simulink model "Kundur_BESS_STA_Nov14_2021a_v2_2021a"  (R2023a)
settings: Solver=VariableStepAuto  StartTime=0.0  StopTime=3  FixedStep=Ts  MaxStep=1e-5  MinStep=1e-20  RelTol=1e-3  EnableMultiTasking=on
PreLoadFcn:
  | Ts=50e-6;
PostLoadFcn:
  | Ts=50e-6;
InitFcn:
  | Ts=50e-6;
values from neighbouring files (symbols this model uses):
  current_K_den = [1 -1.95396088137 0.953960881373]    [param_cntrl_v2.mat]
  current_K_num = [292.549944556 -582.765243791 290.215658722]    [param_cntrl_v2.mat]
  flt_den = [1 -1.99914493247 0.999500180349]    [param_cntrl_v2.mat]
  flt_num = [0.000249925443627 3.12366678454e-08 -0.000249894206959]    [param_cntrl_v2.mat]
  flt_rocof_den = [1 -3.94812243331 5.84544117496 -3.84650440967 0.949185710471]    [param_cntrl_v2.mat]
  flt_rocof_num = [2.65341753303e-09 1.06136701321e-08 1.59205051982e-08 1.06136701321e-08 2.65341753303e-09]    [param_cntrl_v2.mat]
  pll_K_den = [1 -1.95396088137 0.953960881373]    [param_cntrl_v2.mat]
  pll_K_num = [1047.77474974 -2078.89023245 1031.12061217]    [param_cntrl_v2.mat]
  sampling_k = 5e-05    [param_cntrl_v2.mat]
undefined symbols (not defined in the file or in its folder): Ad2, Ad4, Bd2, Bd4, Cd2, Cd4, D1, Delta, flt_rocof_a_den, flt_rocof_a_num, flt_rocof_b_den, flt_rocof_b_num, Gd2, Gd4, Kd2, Kd4, L, R
libraries: spsThreePhaseVIMeasurementLib x15, spsLoadFlowBusLib x12, spsSeriesRLCBranchLib x11, spsThreePhaseSeriesRLCLoadLib x11, spsThreePhaseTransformerTwoWindingsLib x8, spsThreePhaseSeriesRLCBranchLib x8, spsabctoAlphaBetaZeroLib x8, spsGenericPowerSystemStabilizerLib x8, spsPowerPositiveSequenceLib x7, spsThreePhaseParallelRLCLoadLib x6, spsPLL3phLib x6, spsGroundLib x6
(part 1 of 4)
Description:
  | Model of a simple control system for use iin training.
settings Model: Creator=Paul Baracos  LastModifiedBy=juang
settings SolverCC: MaxConsecutiveZCs=10000  MaxConsecutiveMinStep=10  SolverJacobianMethodControl=FullAnalytical
settings DataIOCC: LimitDataPoints=on  SaveFormat=Array  SignalLoggingSaveFormat=ModelDataLogs  SaveOutput=off  SaveTime=off  ReturnWorkspaceOutputs=off  SignalLoggingName=sigsOut
settings OptimizationCC: BlockReduction=off  BooleanDataType=off  OptimizeBlockIOStorage=off  BufferReuse=off  GlobalBufferReuse=off  ExpressionFolding=off  LocalBlockOutputs=off  InitFltsAndDblsToZero=on  LifeSpan=inf  OptimizeDataStoreBuffers=off  BusAssignmentInplaceUpdate=off
settings DebuggingCC: SaveWithParameterizedLinksMsg=none  UnderspecifiedInitializationDetection=Classic  MergeDetectMultiDrivingBlocksExec=none  SignalResolutionControl=TryResolveAllWithWarning  MultiTaskDSMMsg=warning  MultiTaskCondExecSysMsg=none  FcnCallInpInsideContextMsg=warning  UnconnectedInputMsg=warning  UnconnectedOutputMsg=warning  UnconnectedLineMsg=warning  SFUnexpectedBacktrackingDiag=warning  SFNoUnconditionalDefaultTransitionDiag=warning  ArithmeticOperatorsInVariantConditions=warning
settings HardwareCC: ProdBitPerPointer=32  ProdBitPerSizeT=32  ProdBitPerPtrDiffT=32  ProdLargestAtomicFloat=None  ProdIntDivRoundTo=Undefined  ProdEndianess=Unspecified  ProdWordSize=32  ProdHWDeviceType=32-bit Generic  TargetBitPerPointer=64  TargetBitPerSizeT=64  TargetBitPerPtrDiffT=64  TargetLongLongMode=on  TargetIntDivRoundTo=Zero  TargetEndianess=LittleEndian  TargetWordSize=64  TargetHWDeviceType=MATLAB Host  ProdEqTarget=off
settings ModelReferenceCC: EnableRefExpFcnMdlSchedulingChecks=on  PropagateSignalLabelsOutOfModel=off
settings SFSimCC: SimUseLocalCustomCode=off  CustomCodeUndefinedFunction=UseInterfaceOnly
settings RTWCC: RTWUseLocalCustomCode=off
settings CodeAppCC: StateflowObjectComments=on
settings GRTTargetCC: TargetFcnLib=ansi_tfl_tmw.mat  TargetLangStandard=C89/C90 (ANSI)  CombineOutputUpdateFcns=off  GRTInterface=on
settings ConfigComp: CovMetricSettings=dw  CovSaveCumulativeToWorkspaceVar=on  CovSaveSingleToWorkspaceVar=on  CovExternalEMLEnable=off
settings SimscapeCC: SimscapeNormalizeSystem=off

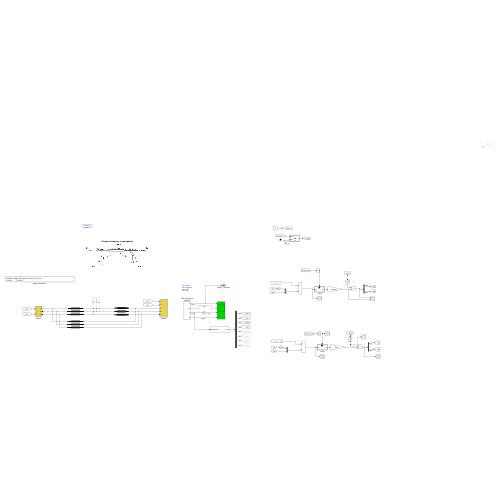
[thumbnail: Simulink's stored preview of the top-level diagram]
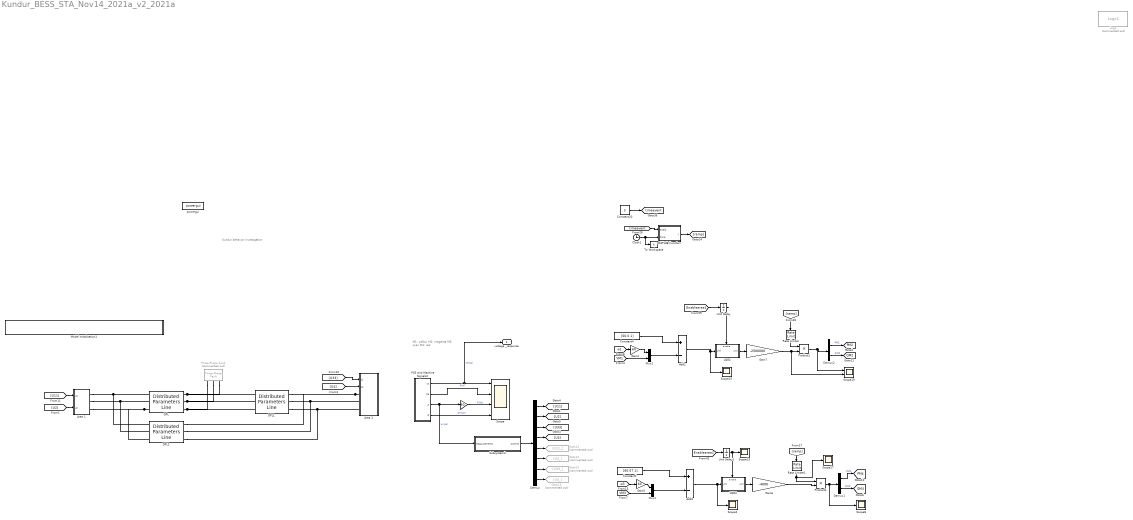
== system Kundur_BESS_STA_Nov14_2021a_v2_2021a ==
  note: Kundur behavior investigation
  note: M1: yellow
      | M2: magenta
      | M3: cyan
      | M4: red
  " " : Gain  Gain=60  SaturateOnIntegerOverflow=on  OutDataTypeStr=Inherit: Same as input  ParamDataTypeStr=Inherit: Same as input
  Add2 : Sum  Inputs=+-
  Add3 : Sum  Inputs=+-
  Area 1 : Subsystem
  Area 2 : Subsystem
  Clock1 : Clock
  Constant1 : Constant  Value=[60.07 1]
  Constant20 : Constant  Value=3
  Constant4 : Constant  Value=[60.0 1]
  DPL : spsDistributedParametersLineLib/Distributed Parameters Line  Phases=3  Length=110  Frequency=60  Resistance=[0.0001*529 1.61]  Inductance=[0.001*529/(377) 0.0061]  Capacitance=[0.00175/529/(377) 5.2489e-9]  x1=[-0.00065 2.34503898169386e-05 162037.072789035 -201564.621940964;-0.0006 2.16068678041118e-05 165807.483999355 -198474.662134838;-0.00055 1.97556689740379e-05 169518.984600121 -195314.185226316;-0.0005 1.78974510488464e-05 173170.255912845 -192084.314117795;-0.00045 1.60328742445181e-05 176760.000658212 -188786.1963671;-0.0004 1.41626010363132e-05 180286.94341701 -185421.003779764;-0.00035 1.22872959233969e-05 183749.831083269 -181989.931992688;-0.0003 1.04076251927465e-05 187147.433309491 -178494.200049342;-0.00025 8.52425668242225e-06 190478.542943782 -174935.04996664;-0.0002 6.63785954428797e-06 193741.976458752 -171313.746293659;-0.00015 4.74910400626456e-06 196936.574372011 -167631.57566235;-0.0001 2.85866113420113e-06 200061.201658132 -163889.846330406;-5e-05 9.67202593448582e-07 203114.74815192 -160089.887716441]  x2=[-0.00065 3.04897605546982e-05 118816.066831868 -195960.878256138;-0.0006 2.90157468011296e-05 122488.530340616 -193686.56156247;-0.00055 2.75314238908845e-05 126117.474257778 -191343.428955741;-0.0005 2.60373191968251e-05 129701.60923686 -188932.312939808;-0.00045 2.45339635672348e-05 133239.661851769 -186454.070172711;-0.0004 2.30218911372104e-05 136730.375049258 -183909.581162304;-0.00035 2.15016391388865e-05 140172.50859555 -181299.749953418;-0.0003 1.99737477105591e-05 143564.839516987 -178625.503806653;-0.00025 1.84387597047774e-05 146906.162534544 -175887.792868933;-0.0002 1.6897220495471e-05 150195.290492063 -173087.589835917;-0.00015 1.53496777841807e-05 153431.054778043 -170225.889606408;-0.0001 1.3796681405463e-05 156612.30574084 -167303.708928874;-5e-05 1.22387831315364e-05 159737.913097136 -164322.086040193]  x3=[-0.00065 -7.70603438254632e-09 386.387902520665 214.266648693801;-0.0006 -8.20654088038672e-09 382.28069114739 221.511346722587;-0.00055 -8.70413163332872e-09 378.037657264824 228.677342824636;-0.0005 -9.19862984974715e-09 373.660308402703 235.762090955653;-0.00045 -9.68985983678033e-09 369.150199812235 242.763073938362;-0.0004 -1.01776470627529e-08 364.508933913525 249.677804356846;-0.00035 -1.06618182191862e-08 359.738159726248 256.503825440312;-0.0003 -1.11422012823736e-08 354.839572283756 263.238711935973;-0.00025 -1.16186255745004e-08 349.814912030842 269.880070970725;-0.0002 -1.2090921824284e-08 344.665964205369 276.425542901327;-0.00015 -1.25589222271158e-08 339.394558203981 282.872802152769;-0.0001 -1.30224605046811e-08 334.00256693213 289.219558044538;-5e-05 -1.3481371964037e-08 328.491906138641 295.463555604487]  x4=[-0.00065 6.9623199876992e-08 236.382256048156 -1248.37836597241;-0.0006 6.7501778785042e-08 259.870303302539 -1243.70107133658;-0.00055 6.53563746325074e-08 283.266019875563 -1238.58189563215;-0.0005 6.3187749671268e-08 306.561093380529 -1233.02265767785;-0.00045 6.09966744034463e-08 329.747247188744 -1227.02533264446;-0.0004 5.87839273076519e-08 352.816243370164 -1220.592051353;-0.00035 5.65502945623917e-08 375.75988562029 -1213.7250995177;-0.0003 5.42965697667444e-08 398.57002217228 -1206.42691693383;-0.00025 5.20235536583985e-08 421.238548693231 -1198.70009661092;-0.0002 4.97320538291541e-08 443.757411163608 -1190.54738385143;-0.00015 4.74228844379892e-08 466.118608738802 -1181.97167527539;-0.0001 4.50968659217932e-08 488.314196591789 -1172.97601779123;-5e-05 4.27548247038692e-08 510.336288735894 -1163.56360751321]  x5=0.000622431770558027  V1=[0 0 0 8.852e-11 2.458e+05 2.458e+05;0 0 0 377 377 377;1.571 1.571 1.571 -1.64 0.7159 -0.8549]  V2=[0 0 0 1.627e-10 2.245e+05 2.245e+05;0 0 0 377 377 377;1.571 1.571 1.571 -1.342 0.5232 -1.048]  I1=[0 0 0 6.584e-13 354.7 354.2;0 0 0 377 377 377;1.571 1.571 1.571 -2.457 2.767 1.197]  I2=[0 0 0 4.221e-13 1404 1403;0 0 0 377 377 377;1.571 1.571 1.571 -0.7538 0.3476 -1.223]  nHarmo=2  Measurements=None  Decoupling=off  VsMag0=0  VrMag0=0  VsAngle0=0  VrAngle0=0  IsMag0=0  IrMag0=0  IsAngle0=0  IrAngle0=0
  DPL1 : spsDistributedParametersLineLib/Distributed Parameters Line  Phases=3  Length=110  Frequency=60  Resistance=[0.0001*529 1.61]  Inductance=[0.001*529/(377) 0.0061]  Capacitance=[0.00175/529/(377) 5.2489e-9]  x1=[-0.00065 3.04897737893273e-05 118816.066831868 -195960.878256138;-0.0006 2.90157601664698e-05 122488.530340616 -193686.56156247;-0.00055 2.75314373821871e-05 126117.474257778 -191343.428955741;-0.0005 2.60373328092966e-05 129701.60923686 -188932.312939808;-0.00045 2.45339772960389e-05 133239.661851769 -186454.070172711;-0.0004 2.30219049774693e-05 136730.375049258 -183909.581162304;-0.00035 2.15016530856827e-05 140172.50859555 -181299.749953418;-0.0003 1.99737617589375e-05 143564.839516987 -178625.503806653;-0.00025 1.84387738497467e-05 146906.162534544 -175887.792868933;-0.0002 1.68972347320055e-05 150195.290492063 -173087.589835917;-0.00015 1.53496921072222e-05 153431.054778043 -170225.889606408;-0.0001 1.37966958099226e-05 156612.30574084 -167303.708928874;-5e-05 1.22387976122963e-05 159737.913097136 -164322.086040193]  x2=[-0.00065 3.28792055379406e-05 73497.1281809996 -185964.418906558;-0.0006 3.18342069047249e-05 76989.2205617754 -184546.068621456;-0.00055 3.07778977293782e-05 80453.9590390789 -183062.149996912;-0.0005 2.97106533135209e-05 83890.1126078269 -181513.190262145;-0.00045 2.86328528440121e-05 87296.4604190179 -179899.739755175;-0.0004 2.75448792582265e-05 90671.7922134945 -178222.371727283;-0.00035 2.64471191079986e-05 94014.908751942 -176481.682139344;-0.0003 2.53399624222828e-05 97324.6222409731 -174678.289450079;-0.00025 2.42238025685775e-05 100599.756755145 -172812.834396324;-0.0002 2.30990361131641e-05 103839.148654759 -170885.979765376;-0.00015 2.19660626802085e-05 107041.646999298 -168898.410159511;-0.0001 2.08252848097767e-05 110206.11395635 -166850.831752747;-5e-05 1.96771078148139e-05 113331.425205873 -164743.972039941]  x3=[-0.00065 -1.95769407602966e-08 351.42047903309 278.927488837443;-0.0006 -1.98750329311255e-08 346.100716190805 285.501615062663;-0.00055 -2.01660635973912e-08 340.657985412057 291.974303923501;-0.0005 -2.04499293572839e-08 335.094220473176 298.343255704425;-0.00045 -2.07265293546507e-08 329.41139815335 304.606207547194;-0.0004 -2.09957653148295e-08 323.611537532293 310.760934254839;-0.00035 -2.12575415795659e-08 317.696699272864 316.805249082269;-0.0003 -2.15117651409993e-08 311.668984888935 322.737004513205;-0.00025 -2.17583456747089e-08 305.530535998722 328.554093023188;-0.0002 -2.19971955718053e-08 299.28353356389 334.254447828369;-0.00015 -2.22282299700572e-08 292.930197114655 339.836043619829;-0.0001 -2.24513667840431e-08 286.472783961208 345.29689728316;-5e-05 -2.26665267343154e-08 279.913588391693 350.635068603058]  x4=[-0.00065 8.49527153453681e-08 55.1658815479513 -1258.43087921918;-0.0006 8.33025259626403e-08 78.8755823413983 -1257.16743857369;-0.00055 8.16227395890926e-08 102.557259016015 -1255.45733232342;-0.0005 7.99139530448253e-08 126.202497584841 -1253.30116806099;-0.00045 7.81767734535609e-08 149.802897007204 -1250.69971186129;-0.0004 7.64118180269363e-08 173.350072173564 -1247.65388800932;-0.00035 7.46197138452107e-08 196.835656884708 -1244.16477867178;-0.0003 7.28010976344665e-08 220.251306824217 -1240.23362351263;-0.00025 7.09566155403837e-08 243.588702523164 -1235.86181925256;-0.0002 6.90869228986678e-08 266.83955231598 -1231.05091917281;-0.00015 6.71926840022114e-08 289.995595286447 -1225.80263256327;-0.0001 6.5274571865075e-08 313.048604202757 -1220.11882411519;-5e-05 6.33332679833675e-08 335.990388440611 -1214.00151325863]  x5=0.000622431770558027  V1=[0 0 0 1.627e-10 2.245e+05 2.245e+05;0 0 0 377 377 377;1.571 1.571 1.571 -1.342 0.5232 -1.048]  V2=[0 0 0 2.11e-10 2.083e+05 2.083e+05;0 0 0 377 377 377;1.571 1.571 1.571 -0.9957 0.2975 -1.273]  I1=[0 0 0 5.999e-13 365.5 365;0 0 0 377 377 377;1.571 1.571 1.571 -1.212 2.93 1.359]  I2=[0 0 0 3.403e-13 1391 1390;0 0 0 377 377 377;1.571 1.571 1.571 2.907 0.203 -1.368]  nHarmo=2  Measurements=None  Decoupling=off  VsMag0=0  VrMag0=0  VsAngle0=0  VrAngle0=0  IsMag0=0  IrMag0=0  IsAngle0=0  IrAngle0=0
  DPL2 : spsDistributedParametersLineLib/Distributed Parameters Line  Phases=3  Length=220  Frequency=60  Resistance=[0.0001*529 1.61]  Inductance=[0.001*529/(377) 0.0061]  Capacitance=[0.00175/529/(377) 5.2489e-9]  x1=[-0.00125 4.47388675144062e-05 112704.215489258 -232770.393652631;-0.0012 4.30375462134881e-05 117071.56879016 -230604.733707614;-0.00115 4.13209338773288e-05 121397.32712012 -228357.140998763;-0.0011 3.95896404101173e-05 125679.953557802 -226028.414085065;-0.00105 3.78442809321789e-05 129917.926506425 -223619.380352103;-0.001 3.60854755614253e-05 134109.74023438 -221130.895718092;-0.00095 3.43138491930299e-05 138253.905410208 -218563.844329773;-0.0009 3.25300312774057e-05 142348.949631757 -215919.138248282;-0.00085 3.07346555965643e-05 146393.417949313 -213197.717125095;-0.0008 2.8928360038936e-05 150385.873382542 -210400.54786818;-0.00075 2.71117863727318e-05 154324.897431037 -207528.624298454;-0.0007 2.52855800179252e-05 158209.090578311 -204582.966796687;-0.00065 2.34503898169386e-05 162037.072789035 -201564.621940964;-0.0006 2.16068678041118e-05 165807.483999355 -198474.662134838;-0.00055 1.97556689740379e-05 169518.984600121 -195314.185226316;-0.0005 1.78974510488464e-05 173170.255912845 -192084.314117795;-0.00045 1.60328742445181e-05 176760.000658212 -188786.1963671;-0.0004 1.41626010363132e-05 180286.94341701 -185421.003779764;-0.00035 1.22872959233969e-05 183749.831083269 -181989.931992688;-0.0003 1.04076251927465e-05 187147.433309491 -178494.200049342;-0.00025 8.52425668242225e-06 190478.542943782 -174935.04996664;-0.0002 6.63785954428797e-06 193741.976458752 -171313.746293659;-0.00015 4.74910400626456e-06 196936.574372011 -167631.57566235;-0.0001 2.85866113420113e-06 200061.201658132 -163889.846330406;-5e-05 9.67202593448582e-07 203114.74815192 -160089.887716441]  x2=[-0.00125 4.44062308903789e-05 29918.4277641747 -197710.675173221;-0.0012 4.35246405678654e-05 33639.6583650254 -197111.626699133;-0.00115 4.26275861478058e-05 37348.9369554381 -196442.54540265;-0.0011 4.17153863493642e-05 41044.945646392 -195703.669005169;-0.00105 4.07883652727854e-05 44726.371263598 -194895.260025957;-0.001 3.98468522842439e-05 48391.905814064 -194017.605688875;-0.00095 3.88911818988212e-05 52040.246950818 -193071.017820329;-0.0009 3.79216936616548e-05 55670.0984356262 -192055.832738482;-0.00085 3.6938732027299e-05 59280.1705995399 -190972.41113376;-0.0008 3.59426462373421e-05 62869.1808011092 -189821.137940699;-0.00075 3.49337901963222e-05 66435.8538820988 -188602.422201184;-0.0007 3.39125223459869e-05 69978.9226205463 -187316.696919113;-0.00065 3.28792055379406e-05 73497.1281809996 -185964.418906558;-0.0006 3.18342069047249e-05 76989.2205617754 -184546.068621456;-0.00055 3.07778977293782e-05 80453.9590390789 -183062.149996912;-0.0005 2.97106533135209e-05 83890.1126078269 -181513.190262145;-0.00045 2.86328528440121e-05 87296.4604190179 -179899.739755175;-0.0004 2.75448792582265e-05 90671.7922134945 -178222.371727283;-0.00035 2.64471191079986e-05 94014.908751942 -176481.682139344;-0.0003 2.53399624222828e-05 97324.6222409731 -174678.289450079;-0.00025 2.42238025685775e-05 100599.756755145 -172812.834396324;-0.0002 2.30990361131641e-05 103839.148654759 -170885.979765376;-0.00015 2.19660626802085e-05 107041.646999298 -168898.410159511;-0.0001 2.08252848097767e-05 110206.11395635 -166850.831752747;-5e-05 1.96771078148139e-05 113331.425205873 -164743.972039941]  x3=[-0.00125 -2.93418450150669e-09 420.706842786539 123.303837466321;-0.0012 -3.36724177725915e-09 418.308051458368 131.211559530522;-0.00115 -3.79910268804167e-09 415.760637271337 139.072662752401;-0.0011 -4.229613795729e-09 413.065505309576 146.884354119415;-0.00105 -4.65862214177452e-09 410.22361314064 154.643858174818;-0.001 -5.08597530155564e-09 407.235970475282 162.348418003767;-0.00095 -5.51152143852959e-09 404.103638808717 169.995296212839;-0.0009 -5.93510935818019e-09 400.82773104347 177.58177590262;-0.00085 -6.35658856173656e-09 397.409411093972 185.105161633;-0.0008 -6.77580929964459e-09 393.849893473024 192.562780380851;-0.00075 -7.19262262477226e-09 390.150442860288 199.951982489743;-0.0007 -7.60688044532988e-09 386.312373652951 207.270142611352;-0.00065 -8.01843557748633e-09 382.337049498727 214.514660638232;-0.0006 -8.42714179766283e-09 378.225882811359 221.682962627624;-0.00055 -8.83285389448545e-09 373.980334268796 228.772501715965;-0.0005 -9.23542772037803e-09 369.601912294218 235.780759023772;-0.00045 -9.63472024277714e-09 365.092172520105 242.705244550597;-0.0004 -1.00305895949509e-08 360.452717235525 249.543498059702;-0.00035 -1.04228951264033e-08 355.68519481685 256.293089952178;-0.0003 -1.08114974528472e-08 350.791299142093 262.951622130164;-0.00025 -1.11962585057263e-08 345.772768989086 269.516728848881;-0.0002 -1.15770415812707e-08 340.631387417694 275.986077557175;-0.00015 -1.19537113890666e-08 335.368981136309 282.357369726252;-0.0001 -1.23261341001251e-08 329.987419852826 288.628341666344;-5e-05 -1.26941773944301e-08 324.488615610343 294.79676533098]  x4=[-0.00125 9.3026611658606e-08 -227.277448411085 -1227.94404256492;-0.0012 9.1902598207341e-08 -204.092223618631 -1232.0096275895;-0.00115 9.0745932200538e-08 -180.834485830935 -1235.63748545975;-0.0011 8.95570245961215e-08 -157.512498411488 -1238.82632721505;-0.00105 8.83362978073024e-08 -134.134547551369 -1241.57501987511;-0.001 8.70841855524961e-08 -110.708939325203 -1243.88258684251;-0.00095 8.58011327012246e-08 -87.2439967400488 -1245.74820824971;-0.0009 8.44875951160566e-08 -63.7480567782751 -1247.17122125028;-0.00085 8.31440394906415e-08 -40.229467435472 -1248.15112025451;-0.0008 8.17709431838955e-08 -16.6965847544464 -1248.68755710892;-0.00075 8.03687940503983e-08 6.84223014363966 -1248.78034122006;-0.0007 7.89380902670605e-08 30.3786140299359 -1248.42943962219;-0.00065 7.74793401561238e-08 53.9042045393185 -1247.63497698896;-0.0006 7.59930620045567e-08 77.4106431414995 -1246.39723558917;-0.00055 7.44797838799093e-08 100.889578110772 -1244.71665518644;-0.0005 7.29400434426936e-08 124.33266749334 -1242.59383288299;-0.00045 7.13743877553554e-08 147.731582071172 -1240.02952290747;-0.0004 6.97833730879053e-08 171.078008321335 -1237.02463634701;-0.00035 6.81675647202788e-08 194.36365136975 -1233.5802408235;-0.0003 6.65275367414951e-08 217.580237938319 -1229.69756011426;-0.00025 6.48638718456858e-08 240.719519284383 -1225.37797371726;-0.0002 6.31771611250668e-08 263.773274131459 -1220.62301636098;-0.00015 6.14680038599256e-08 286.733311590223 -1215.43437745912;-0.0001 5.97370073057e-08 309.591474068694 -1209.8139005104;-5e-05 5.79847864772236e-08 332.339640170585 -1203.76358244349]  x5=0.00124486354111605  V1=[0 0 0 8.852e-11 2.458e+05 2.458e+05;0 0 0 377 377 377;1.571 1.571 1.571 -1.875 0.5704 -1]  V2=[0 0 0 2.11e-10 2.083e+05 2.083e+05;0 0 0 377 377 377;1.571 1.571 1.571 -1.23 0.152 -1.419]  I1=[0 0 0 4.126e-13 353.3 352.8;0 0 0 377 377 377;1.571 1.571 1.571 -1.923 2.627 1.056]  I2=[0 0 0 9.94e-14 1379 1379;0 0 0 377 377 377;1.571 1.571 1.571 1.346 0.05721 -1.513]  nHarmo=2  Measurements=None  Decoupling=off  VsMag0=0  VrMag0=0  VsAngle0=0  VrAngle0=0  IsMag0=0  IrMag0=0  IsAngle0=0  IrAngle0=0
  Demux : Demux  Outputs=8
  Demux1 : Demux  Outputs=2
  Demux2 : Demux  Outputs=2
  Gain4 : Gain  Gain=60
  Gain5 : Gain  Gain=60
  Gain6 : Gain  Gain=-4000
  Gain7 : Gain  Gain=-2500000
  Goto12 : Goto  Commented=on  GotoTag=U2_
  Goto13 : Goto  Commented=on  GotoTag=U4_
  Goto14 : Goto  Commented=on  GotoTag=U11_
  Goto15 : Goto  Commented=on  GotoTag=U33_
  LQG2 : Subsystem
  LQG4 : Subsystem
  Logo : opal_lib/Logo1  Commented=on  vide=[]
  MATLAB Function : MATLAB Function  TreatAsAtomicUnit=on
  Model Initialization1 : Subsystem  mask(Model Functions){InitFcnX=Ts=50e-6;, prel=on, posl=on, inif=on, strf=off}
      mask prompts: InitFcnX "Initialisation"; prel "Preload Function"; posl "PostLoad Function"; inif "InitFcn"; strf "StartFcn"
      mask init:
      | currentBlock = gcb;
      | root = bdroot(currentBlock);
      | 
      | if ~strcmp(get_param(root,'BlockDiagramType'),'library')
      |     if prel==1
      |         set_param(root, 'PreLoadFcn', InitFcnX);
      |     else
      |         set_param(root, 'PreLoadFcn', '');
      |     end
      |     if inif==1
      |         set_param(root, 'InitFcn', InitFcnX);
      |     else
      |         set_param(root, 'InitFcn', '');
      |     end
      |     if strf==1
      |         set_param(root, 'StartFcn', InitFcnX);
      |     else
      |         set_param(root, 'StartFcn', '');
      |     end
      |     if posl==1
      |         set_param(root, 'PostLoadFcn', InitFcnX);
      |     else
      |         set_param(root, 'PostLoadFcn', '');
      |     end
      | end
      | 
      | pos = get_param(currentBlock, 'Position');
      | width = pos(3) - pos(1); height = pos(4) - pos(2);
      | txt = [ upper(root) '\n' '- InitFcn. . . . . '  get_param(root, 'InitFcn') ];
      settings: CopyFcn=set_param(gcb,'LinkStatus','none')
      mask Display: text(5, height*0.5, txt, 'horizontalAlignment', 'left', 'verticalAlignment', 'middle') ;
  Mux1 : Mux  Inputs=2
  Mux2 : Mux  Inputs=2
  PSS and Machine Signals2 : Subsystem
  Product1 : Product
  Product2 : Product
  Rate Limiter : RateLimiter  RisingSlewLimit=0.02  FallingSlewLimit=-0.02  SampleTimeMode=inherited  InitialCondition=1
  Rate Limiter1 : RateLimiter  RisingSlewLimit=0.02  FallingSlewLimit=-0.02  SampleTimeMode=inherited  InitialCondition=1
  Scope : Scope  NumInputPorts=4
  Scope{2,8,13,15,17} (5 alike) : Scope
  Scope19 : Scope  NumInputPorts=2
  Subsystem3 : Subsystem
  Three-Phase Fault : spsThreePhaseFaultLib/Three-Phase Fault  Commented=on  InitialStates=0  FaultA=on  FaultB=on  FaultC=on  GroundFault=off  SwitchTimes=[ 5 5.05 ]  External=off  SwitchStatus=NaN  FaultResistance=0.0001  GroundResistance=100  SnubberResistance=1e6  SnubberCapacitance=inf  Measurements=None
  To Workspace : ToWorkspace  VariableName=t  SampleTime=Ts
      settings: Save2DSignal=2-D array (concatenate along first dimension)
  Unit Delay : UnitDelay  SampleTime=-1  HasFrameUpgradeWarning=on
  Unit Delay1 : UnitDelay  SampleTime=-1  HasFrameUpgradeWarning=on
  powergui : spspowerguiLib/powergui  Priority=2  SimulationMode=Discrete  SampleTime=Ts  frequency=60  Iterations=50  frequencyindice=0  Pbase=100e6  ErrMax=1e-4  UnitsV=kV  UnitsW=MW  buscounter=0  FunctionMessages=off  echomessages=off  EnableUseOfTLC=off  CurrentSourceSwitches=off  DisableSnubberDevices=off  DisableRonSwitches=off  DisableVfSwitches=off  DisplayEquations=off  AutomaticDiscreteSolvers=off  SolverType=Tustin  Interpol=off  ExternalGateDelay=off  methode=off  Ts=0  x0status=blocks  SPID=off  SwTol=0  HookPort=off  NonlinearTolerance=0  nMaxIteration=15  ContinueOnMaxIteration=off  RestoreLinks=warning  ResistiveCurrentMeasurement=off  Frange=logspace(0,3,50)  Ylog=off  Xlog=off  ShowGrid=off  save=off  variable=ZData  structure=0  ZoomFFT=on  StartTime=0.0  cycles=1  DisplayStyle=1  fundamental=60  FreqAxis=off  MaxFrequency=1000  frequencyindicesteady=1  RmsSteady=1  display=off
  voltage _response : Outport  VectorParamsAs1DForOutWhenUnconnected=off
  tag scope: PM2=global, PM4=global, QM2=global, QM4=global, timeevent=global
  wires:
  Demux1/1 -> [PM4]  "PM2"
  Unit Delay1/1 -> LQG4/Enable, Scope13/1
  [timeevent] -> MATLAB Function/1(event)
  Unit Delay/1 -> LQG2/Enable
  Gain7/1 -> Scope19/2, Product1/2
  [Enablearea2] -> Unit Delay1/1
  Demux/4 -> [U4]
  Demux/6 -> Goto12/1
  Mux2/1 -> Add2/2
  Demux1/2 -> [QM4]  "QM2"
  [w3] -> Gain5/1
  Rate Limiter1/1 -> Scope17/1, Product2/1
  Demux/7 -> Goto15/1
  [Enablearea1] -> Unit Delay/1
  Demux/3 -> [U33]
  MATLAB Function/1(y) -> [ramp]
  Gain6/1 -> Product2/2
  PSS and Machine Signals2/2("Pe ") -> Scope/2  "P(w)"
  Product2/1 -> Scope8/1, Demux1/1
  Gain4/1 -> Mux2/1
  Subsystem3/1(Control) -> Demux/1
  Rate Limiter/1 -> Product1/1
  PSS and Machine Signals2/3(w) -> Subsystem3/1(Measurements), " "/1  "w (pu)"
  Demux/5 -> Goto14/1
  Demux/8 -> Goto13/1
  Constant4/1 -> Add2/1
  Constant20/1 -> [timeevent]
  [VM1] -> Mux2/2
  PSS and Machine Signals2/4(Q) -> Scope/4  "Q(VAr)"
  [U4] -> Area 2/2(u2)
  Constant1/1 -> Add3/1
  " "/1 -> Scope/3  "f (Hz)"
  Gain5/1 -> Mux1/1
  Mux1/1 -> Add3/2
  [U11] -> Area 1/1(u1)
  Clock1/1 -> To Workspace/1, MATLAB Function/2(time)
  [VM3] -> Mux1/2
  [ramp] -> Rate Limiter/1
  Demux2/1 -> [PM2]  "PM2"
  Add3/1 -> Scope2/1, LQG4/1(y(t))
  Product1/1 -> Scope19/1, Demux2/1
  [U33] -> Area 2/1(u1)
  [U2] -> Area 1/2(u2)
  LQG2/1(u(t)) -> Gain7/1
  [w1] -> Gain4/1
  LQG4/1(u(t)) -> Gain6/1
  Demux/1 -> [U11]
  PSS and Machine Signals2/1(Vt) -> voltage _response/1, Scope/1  "Vt(pu)"
  Add2/1 -> Scope15/1, LQG2/1(y(t))
  Demux2/2 -> [QM2]  "QM2"
  Demux/2 -> [U2]
  [ramp] -> Rate Limiter1/1
  connections:
  DPL/LConn3 -- DPL2/LConn3 -- Area 1/RConn3
  DPL/RConn1 -- Three-Phase Fault/LConn1 -- DPL1/LConn1
  DPL/RConn3 -- Three-Phase Fault/LConn3 -- DPL1/LConn3
  Area 2/LConn1 -- DPL2/RConn1 -- DPL1/RConn1
  Area 1/RConn2 -- DPL2/LConn2 -- DPL/LConn2
  DPL1/RConn3 -- DPL2/RConn3 -- Area 2/LConn3
  DPL1/RConn2 -- DPL2/RConn2 -- Area 2/LConn2
  DPL/RConn2 -- Three-Phase Fault/LConn2 -- DPL1/LConn2
  Area 1/RConn1 -- DPL2/LConn1 -- DPL/LConn1

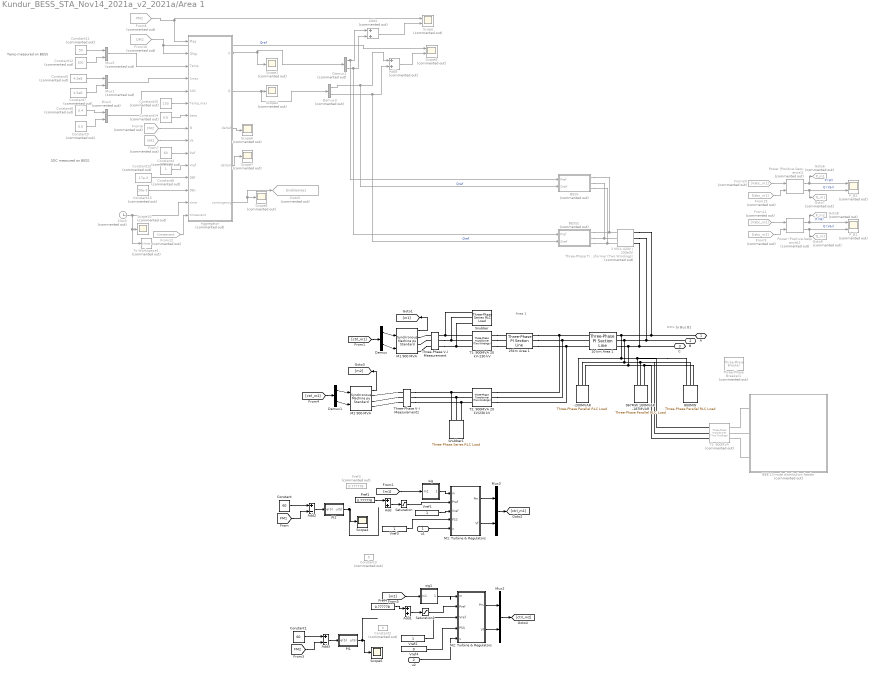
== system Kundur_BESS_STA_Nov14_2021a_v2_2021a/Area 1 ==
  note: Temp measured on BESS
  note: Area 1
  note: ==> to Bus B1
  note: SOC measured on BESS
  u1 : Inport
  u2 : Inport  Port=2
  -200MVAR : spsThreePhaseParallelRLCLoadLib/Three-Phase Parallel RLC Load  LConnTagsString=A|B|C  Configuration=Y (grounded)  NominalVoltage=230e3  Vabc=[1e3 1e3 1e3]  Vabcp=[1e3 1e3 1e3]  NominalFrequency=60  UnbalancedPower=off  ActivePower=0  InductivePower=0  CapacitivePower=200e6  Pabc=[10e3 9e3 11e3]  QLabc=[100 90 110]  QCabc=[100 90 110]  Pabcp=[10e3 9e3 11e3]  QLabcp=[100 90 110]  QCabcp=[100 90 110]  Measurements=None  LoadType=constant Z
  10 km Area 1 : spsThreePhasePISectionLineLib/Three-Phase PI Section Line  LConnTagsString=a|b|c  RConnTagsString=A|B|C  Length=10  Frequency=60  Resistances=[0.0001*529 1.61]  Inductances=[0.001*529/(377) 0.0061]  Capacitances=[0.00175/529/(377) 5.2489e-9]
  2 MVA 420V / 230e3V : spsThreePhaseTransformerTwoWindingsLib/Three-Phase Transformer (Two Windings)  Commented=on  Winding1Connection=Delta (D1)  Winding2Connection=Yg  CoreType=Three single-phase transformers  SetSaturation=off  Hysteresis=off  DataFile='hysteresis'  SetInitialFlux=off  Measurements=None  UNITS=pu  NominalPower=[900e6 , 60 ]  Winding1=[ 230e3 , 0.001 , 0.03 ]  Winding2=[ 420 , 0.001 , 0.03 ]  Rm=500  Lm=500  L0=0.5  Saturation=[ 0,0 ; 0.0024,1.2 ; 1.0,1.52 ]  InitialFluxes=[0.79999 -0.79999 0.7]  BreakLoop=off  DiscreteSolver=Trapezoidal iterative  DataType=off  TransfoNumber=0
  25km Area 1 : spsThreePhasePISectionLineLib/Three-Phase PI Section Line  LConnTagsString=a|b|c  RConnTagsString=A|B|C  Length=25  Frequency=60  Resistances=[0.0001*529 1.61]  Inductances=[0.001*529/(377) 0.0061]  Capacitances=[0.00175/529/(377) 5.2489e-9]
  "800MW " : spsThreePhaseParallelRLCLoadLib/Three-Phase Parallel RLC Load  LConnTagsString=A|B|C  Configuration=Y (grounded)  NominalVoltage=230e3  Vabc=[1e3 1e3 1e3]  Vabcp=[1e3 1e3 1e3]  NominalFrequency=60  UnbalancedPower=off  ActivePower=50e6  InductivePower=50e6  CapacitivePower=0  Pabc=[10e3 9e3 11e3]  QLabc=[100 90 110]  QCabc=[100 90 110]  Pabcp=[10e3 9e3 11e3]  QLabcp=[100 90 110]  QCabcp=[100 90 110]  Measurements=None  LoadType=constant Z
  967MW 100MVAR -187MVAR : spsThreePhaseParallelRLCLoadLib/Three-Phase Parallel RLC Load  LConnTagsString=A|B|C  Configuration=Y (grounded)  NominalVoltage=230e3  Vabc=[1e3 1e3 1e3]  Vabcp=[1e3 1e3 1e3]  NominalFrequency=60  UnbalancedPower=off  ActivePower=967e6  InductivePower=100e6  CapacitivePower=187e6  Pabc=[10e3 9e3 11e3]  QLabc=[100 90 110]  QCabc=[100 90 110]  Pabcp=[10e3 9e3 11e3]  QLabcp=[100 90 110]  QCabcp=[100 90 110]  Measurements=None  LoadType=constant Z
  Add : Sum
  Add1 : Sum
  Add2 : Sum  Inputs=+-
  Add3 : Sum  Inputs=+-
  Add4 : Sum  Commented=on
  Add5 : Sum  Commented=on
  Aggregator : MATLAB Function  Commented=on  TreatAsAtomicUnit=on
  BESS : Subsystem  Commented=on  mask(Off-board charger for EVs){Kp=1, Ki=5, C=3600e-6, Vdc=800, Ts=Ts}
      mask prompts: Kp "Current Controller Kp"; Ki "Current Controller Ki"; C "DC link capacitor [uF]"; Vdc "DC link voltage level [V]"; Ts "Sample period [s]"
      mask help: This model only contains the three phase inverter and current controllers in rotating reference frame (PQ). The DAB converter need to be completed. It only has the inverter to improve the simulation time.
      mask Display: image('parking_lot3.png');
  "BESS2 " : Subsystem  Commented=on  mask(Off-board charger for EVs){Kp=1, Ki=5, C=3600e-6, Vdc=800, Ts=Ts}
      mask prompts: Kp "Current Controller Kp"; Ki "Current Controller Ki"; C "DC link capacitor [uF]"; Vdc "DC link voltage level [V]"; Ts "Sample period [s]"
      mask help: This model only contains the three phase inverter and current controllers in rotating reference frame (PQ). The DAB converter need to be completed. It only has the inverter to improve the simulation time.
      mask Display: image('parking_lot3.png');
  Clock : Clock  Commented=on
  Constant : Constant  Value=60
  Constant1 : Constant  Value=60
  Constant10 : Constant  Commented=on  Value=150
  Constant11 : Constant  Commented=on  Value=50
  Constant12 : Constant  Commented=on  Value=100
  Constant13 : Constant  Commented=on  Value=17e-3
  Constant14 : Constant  Commented=on  Value=0.6
  Constant15 : Constant  Commented=on  Value=50e-3
  Constant2 : Constant  Commented=on  Value=0
  Constant3 : Constant  Commented=on  Value=0
  Constant4 : Constant  Commented=on  Value=60
  Constant5 : Constant  Commented=on  Value=4.5e8
  Constant6 : Constant  Commented=on
  Constant7 : Constant  Commented=on  Value=4.5e8
  Constant8 : Constant  Commented=on  Value=0.4
  Constant9 : Constant  Commented=on  Value=0.6
  Demux : Demux  Outputs=[1 1]
  Demux1 : Demux  Outputs=[1 1]
  Demux2 : Demux  Commented=on  Outputs=2
  Demux3 : Demux  Commented=on  Outputs=2
  From10 : From  Commented=on  GotoTag=QM2  TagVisibility=global
  From11 : From  Commented=on  GotoTag=Vabc_m2  TagVisibility=global
      settings: CloseFcn=tagdialog Close
  From12 : From  Commented=on  GotoTag=timeevent  TagVisibility=global
  From19 : From  Commented=on  GotoTag=Iabc_m1  TagVisibility=global
      settings: CloseFcn=tagdialog Close
  From20 : From  Commented=on  GotoTag=Vabc_m1  TagVisibility=global
      settings: CloseFcn=tagdialog Close
  From6 : From  Commented=on  GotoTag=FM2  TagVisibility=global
  From7 : From  Commented=on  GotoTag=VM2  TagVisibility=global
  From8 : From  Commented=on  GotoTag=PM2  TagVisibility=global
  From9 : From  Commented=on  GotoTag=Iabc_m2  TagVisibility=global
      settings: CloseFcn=tagdialog Close
  Goto5 : Goto  Commented=on  GotoTag=Enablearea1  TagVisibility=global
  Goto6 : Goto  Commented=on  GotoTag=P_m1  TagVisibility=global
  Goto7 : Goto  Commented=on  GotoTag=Q_m1  TagVisibility=global
  Goto8 : Goto  Commented=on  GotoTag=P_m2  TagVisibility=global
  Goto9 : Goto  Commented=on  GotoTag=Q_m2  TagVisibility=global
  IEEE 13-node distribution feeder : Subsystem  Commented=on
  M1 900 MVA : spsSynchronousMachinepuStandardLib/Synchronous Machine pu Standard  PresetModel=No  MechanicalLoad=Mechanical power Pm  ShowDetailedParameters=on  RotorType=Round  Units=per unit standard parameters  MeasurementBus=off  NominalParameters="[900E6  20000   60 ]"  Reactances1=[1.8 .3 .25 1.7 .55 .25 .2]  Reactances2=[ 1.305, 0.296, 0.252, 0.474, 0.243, 0.18 ]  dAxisTimeConstants=Open-circuit  qAxisTimeConstants=Open-circuit  TimeConstants1=[]  TimeConstants2=[8 .03 .4 .05]  TimeConstants3=[]  TimeConstants4=[]  TimeConstants5=[ 1.01, 0.053, 0.1 ]  TimeConstants6=[]  TimeConstants7=[]  TimeConstants8=[]  StatorResistance=0.0025  Mechanical="[ 6.5 0  4]"  PolePairs=4  InitialConditions=[0 -31.4247 0.784453 0.784453 0.784453 2.7401 -117.26 122.74 1.83395]  SetSaturation=off  Saturation=[0.6404,0.7127,0.8441,0.9214,0.9956,1.082,1.19,1.316,1.457;0.7,0.7698,0.8872,0.9466,0.9969,1.046,1.1,1.151,1.201]  LoadFlowParameters=[1 700000000 0 0 0]  TsPowergui=0  TsBlock=-1  IterativeModel=Trapezoidal non iterative  IterativeDiscreteModel=Trapezoidal non iterative  BusType=PV  Pref=700000000  Qref=0  Qmin=-inf  Qmax=inf  PLF=0  QLF=0
  M1: Turbine & Regulators : Subsystem
  M2 900 MVA : spsSynchronousMachinepuStandardLib/Synchronous Machine pu Standard  PresetModel=No  MechanicalLoad=Mechanical power Pm  ShowDetailedParameters=on  RotorType=Round  Units=per unit standard parameters  MeasurementBus=off  NominalParameters="[900E6  20000   60 ]"  Reactances1=[1.8 .3 .25 1.7 .55 .25 .2]  Reactances2=[ 1.305, 0.296, 0.252, 0.474, 0.243, 0.18 ]  dAxisTimeConstants=Open-circuit  qAxisTimeConstants=Open-circuit  TimeConstants1=[]  TimeConstants2=[8 .03 .4 .05]  TimeConstants3=[]  TimeConstants4=[]  TimeConstants5=[ 1.01, 0.053, 0.1 ]  TimeConstants6=[]  TimeConstants7=[]  TimeConstants8=[]  StatorResistance=0.0025  Mechanical="[ 6.5 0  4]"  PolePairs=4  InitialConditions=[0 -42.8075 0.788608 0.788608 0.788608 -9.54571 -129.546 110.454 1.86756]  SetSaturation=off  Saturation=[0.6404,0.7127,0.8441,0.9214,0.9956,1.082,1.19,1.316,1.457;0.7,0.7698,0.8872,0.9466,0.9969,1.046,1.1,1.151,1.201]  LoadFlowParameters=[2 700000000 0 0 0]  TsPowergui=0  TsBlock=-1  IterativeModel=Trapezoidal non iterative  IterativeDiscreteModel=Trapezoidal non iterative  BusType=swing  Pref=0  Qref=0  Qmin=-inf  Qmax=inf  PLF=0  QLF=0
  M2: Turbine & Regulators : Subsystem
  Mux1 : Mux  Commented=on  Inputs=2
  Mux2 : Mux  Inputs=2
  Mux3 : Mux  Inputs=2
  Mux4 : Mux  Commented=on  Inputs=2
  Mux5 : Mux  Commented=on  Inputs=2
  PI1 : Subsystem
  PI2 : Subsystem
  P_B1 : Scope  Commented=on  NumInputPorts=2
  P_B2 : Scope  Commented=on  NumInputPorts=2
  Power (Positive-Sequence)1 : spsPowerPositiveSequenceLib/Power (Positive-Sequence)  Commented=on  Freq=60  Vinit=[0, 0]  Iinit=[0, 0]  Ts=Ts
  Power (Positive-Sequence)2 : spsPowerPositiveSequenceLib/Power (Positive-Sequence)  Commented=on  Freq=60  Vinit=[0, 0]  Iinit=[0, 0]  Ts=Ts
  Pref1 : Constant  Value=0.777778
  Pref3 : Constant  Commented=on  Value=0.777778
  Pref4 : Constant  Value=0.777778
  Saturation : Saturate  UpperLimit=1  LowerLimit=0
  Saturation1 : Saturate  UpperLimit=1  LowerLimit=0
  Scope : Scope  Commented=on  NumInputPorts=2
  Scope{1..2,6..8,10} (6 alike) : Scope  Commented=on
  Scope4 : Scope
  Scope5 : Scope
  Scope9 : Scope  Commented=on  NumInputPorts=2
  Snubber : spsThreePhaseSeriesRLCLoadLib/Three-Phase Series RLC Load  LConnTagsString=A|B|C  Configuration=Y (grounded)  NominalVoltage=20000  Vabc=[1e3 1e3 1e3]  Vabcp=[1e3 1e3 1e3]  NominalFrequency=60  UnbalancedPower=off  ActivePower=1e6  InductivePower=0  CapacitivePower=1e7  Pabc=[10e3 9e3 11e3]  QLabc=[100 90 110]  QCabc=[100 90 110]  Pabcp=[10e3 9e3 11e3]  QLabcp=[100 90 110]  QCabcp=[100 90 110]  Measurements=None  LoadType=constant Z
  Snubber1 : spsThreePhaseSeriesRLCLoadLib/Three-Phase Series RLC Load  LConnTagsString=A|B|C  Configuration=Y (grounded)  NominalVoltage=20000  Vabc=[1e3 1e3 1e3]  Vabcp=[1e3 1e3 1e3]  NominalFrequency=60  UnbalancedPower=off  ActivePower=1e6  InductivePower=0  CapacitivePower=1e7  Pabc=[10e3 9e3 11e3]  QLabc=[100 90 110]  QCabc=[100 90 110]  Pabcp=[10e3 9e3 11e3]  QLabcp=[100 90 110]  QCabcp=[100 90 110]  Measurements=None  LoadType=constant Z
  "T1: 900MVA " : spsThreePhaseTransformerTwoWindingsLib/Three-Phase Transformer (Two Windings)  Commented=on  Winding1Connection=Delta (D1)  Winding2Connection=Yg  CoreType=Three single-phase transformers  SetSaturation=off  Hysteresis=off  DataFile='hysteresis'  SetInitialFlux=off  Measurements=None  UNITS=pu  NominalPower="[ 900e6   60 ]"  Winding1="[ 4160  1e-6   0  ]"  Winding2="[ 230e3  1e-6   0.15 ]"  Rm=500  Lm=500  L0=0.5  Saturation="[ 0,0  ;  0.005,1.2  ;  1.0,1.4 ]"  InitialFluxes=[ 0.8 , -0.8 , 0.7 ]  BreakLoop=off  DiscreteSolver=Trapezoidal iterative  DataType=off  TransfoNumber=0
  T1: 900MVA 20 kV-230 kV : spsThreePhaseTransformerTwoWindingsLib/Three-Phase Transformer (Two Windings)  Winding1Connection=Delta (D1)  Winding2Connection=Yg  CoreType=Three single-phase transformers  SetSaturation=off  Hysteresis=off  DataFile='hysteresis'  SetInitialFlux=off  Measurements=None  UNITS=pu  NominalPower="[ 900e6   60 ]"  Winding1="[ 20e3  1e-6   0  ]"  Winding2="[ 230e3  1e-6   0.15 ]"  Rm=500  Lm=500  L0=0.5  Saturation="[ 0,0  ;  0.005,1.2  ;  1.0,1.4 ]"  InitialFluxes=[ 0.8 , -0.8 , 0.7 ]  BreakLoop=off  DiscreteSolver=Trapezoidal iterative  DataType=off  TransfoNumber=0
  T2: 900MVA 20 kV/230 kV : spsThreePhaseTransformerTwoWindingsLib/Three-Phase Transformer (Two Windings)  Winding1Connection=Delta (D1)  Winding2Connection=Yg  CoreType=Three single-phase transformers  SetSaturation=off  Hysteresis=off  DataFile='hysteresis'  SetInitialFlux=off  Measurements=None  UNITS=pu  NominalPower=[ 900e6 60 ]  Winding1="[ 20e3 1e-6  0.0]"  Winding2=[ 230e3 1e-6 0.15]  Rm=500  Lm=500  L0=0.5  Saturation="[ 0,0  ;  0.005,1.2  ;  1.0,1.4 ]"  InitialFluxes=[ 0.8 , -0.8 , 0.7 ]  BreakLoop=off  DiscreteSolver=Trapezoidal iterative  DataType=off  TransfoNumber=0
  Three-Phase V-I Measurement : spsThreePhaseVIMeasurementLib/Three-Phase V-I Measurement  VoltageMeasurement=phase-to-ground  SetLabelV=on  LabelV=Vabc_m1  Vpu=off  VpuLL=off  CurrentMeasurement=yes  SetLabelI=on  LabelI=Iabc_m1  Ipu=off  Pbase=100e6  Vbase=500e3  OutputType=Complex  PhasorSimulation=off  PSBequivalent=0
  Three-Phase V-I Measurement1 : spsThreePhaseVIMeasurementLib/Three-Phase V-I Measurement  VoltageMeasurement=phase-to-ground  SetLabelV=on  LabelV=Vabc_m2  Vpu=off  VpuLL=off  CurrentMeasurement=yes  SetLabelI=on  LabelI=Iabc_m2  Ipu=off  Pbase=100e6  Vbase=500e3  OutputType=Complex  PhasorSimulation=off  PSBequivalent=0
  Three-Phase Breaker1 : spsThreePhaseBreakerLib/Three-Phase Breaker  Commented=on  InitialState=open  SwitchA=on  SwitchB=on  SwitchC=on  SwitchTimes=[1.5]  External=off  BreakerResistance=0.01  SnubberResistance=1e6  SnubberCapacitance=inf  Measurements=None
  To Workspace1 : ToWorkspace  Commented=on  VariableName=time  SampleTime=Ts
      settings: Save2DSignal=2-D array (concatenate along first dimension)
  Vref1 : Constant
  Vref2 : Constant
  Vref3 : Constant
  Vref4 : Constant  Value=0
  sig : Subsystem
  sig1 : Subsystem
  " A" : PMIOPort  Side=Right
  " B" : PMIOPort  Port=2  Side=Right
  " C" : PMIOPort  Port=3  Side=Right
  wires:
  [ctrl_m1] -> Demux/1
  Demux/1 -> M1 900 MVA/1
  Demux/2 -> M1 900 MVA/2
  Vref2/1 -> M2: Turbine & Regulators/3(Vref)
  M2: Turbine & Regulators/2(Vf) -> Mux2/2
  M2: Turbine & Regulators/1(Pm) -> Mux2/1
  M1: Turbine & Regulators/1(Pm) -> Mux3/1
  M1: Turbine & Regulators/2(Vf) -> Mux3/2
  Vref4/1 -> M2: Turbine & Regulators/4(PSS)
  sig/1(Out1) -> M1: Turbine & Regulators/1(m)
  M1 900 MVA/1 -> [m1]
  M2 900 MVA/1 -> [m2]
  [m1] -> sig/1(In1)
  Vref3/1 -> M1: Turbine & Regulators/4(PSS)
  Mux3/1 -> [ctrl_m1]
  Mux2/1 -> [ctrl_m2]
  [ctrl_m2] -> Demux1/1
  Demux1/1 -> M2 900 MVA/1
  Demux1/2 -> M2 900 MVA/2
  sig1/1(Out1) -> M2: Turbine & Regulators/1(m)
  [m2] -> sig1/1(In1)
  Vref1/1 -> M1: Turbine & Regulators/3(Vref)
  u1/1 -> M1: Turbine & Regulators/5(u)
  u2/1 -> M2: Turbine & Regulators/5(u)
  Demux2/2 -> "BESS2 "/1(Pref), Add4/2
  Demux3/2 -> "BESS2 "/2(Qref), Add5/2  "Qref"
  Pref1/1 -> Add/1
  Add/1 -> Saturation/1
  Saturation/1 -> M1: Turbine & Regulators/2(Pref)
  Add1/1 -> Saturation1/1
  Saturation1/1 -> M2: Turbine & Regulators/2(Pref)
  Pref4/1 -> Add1/1
  Add2/1 -> PI2/1(e(S))
  Constant7/1 -> Mux1/2
  Constant5/1 -> Mux1/1
  Mux1/1 -> Aggregator/4(Smax)
  Constant8/1 -> Mux4/1
  Constant9/1 -> Mux4/2
  Mux4/1 -> Aggregator/5(SOC)
  Mux5/1 -> Aggregator/3(Temp)
  Constant11/1 -> Mux5/1
  Constant12/1 -> Mux5/2
  Constant10/1 -> Aggregator/6(Temp_max)
  Constant14/1 -> Aggregator/7(beta)
  Aggregator/1(P) -> Scope1/1, Demux2/1
  From8/1 -> Scope/1, Aggregator/1(Plqg)
  From10/1 -> Scope9/1, Aggregator/2(Qlqg)  "Qref"
  PI2/1(u(S)) -> Scope4/1
  PI1/1(u(S)) -> Scope5/1
  [FM1] -> Add2/2
  Constant/1 -> Add2/1
  [FM2] -> Add3/2
  Constant1/1 -> Add3/1
  Add3/1 -> PI1/1(e(S))
  From6/1 -> Aggregator/8(fk)
  From7/1 -> Aggregator/9(Vk)
  Constant4/1 -> Aggregator/10(fref)
  Constant6/1 -> Aggregator/11(Vref)
  Constant13/1 -> Aggregator/12(DBf)
  Constant15/1 -> Aggregator/13(DBv)
  Aggregator/3(deltaf) -> Scope6/1
  Aggregator/4(deltaV) -> Scope7/1
  Demux2/1 -> BESS/1(Pref), Add4/1
  Demux3/1 -> BESS/2(Qref), Add5/1  "Qref"
  Aggregator/5(contingency) -> Goto5/1, Scope8/1
  Add4/1 -> Scope/2
  Add5/1 -> Scope9/2
  Clock/1 -> Aggregator/14(time), To Workspace1/1, Scope10/1
  From19/1 -> Power (Positive-Sequence)1/2
  From20/1 -> Power (Positive-Sequence)1/1
  Power (Positive-Sequence)1/1 -> Goto6/1, P_B2/1  "P (W)"
  Power (Positive-Sequence)1/2 -> Goto7/1, P_B2/2  "Q (Var)"
  From11/1 -> Power (Positive-Sequence)2/1
  From9/1 -> Power (Positive-Sequence)2/2
  Power (Positive-Sequence)2/2 -> Goto9/1, P_B1/2  "Q (Var)"
  Power (Positive-Sequence)2/1 -> Goto8/1, P_B1/1  "P (W)"
  From12/1 -> Aggregator/15(timeevent)
  Aggregator/2(Q) -> Demux3/1, Scope2/1
  connections:
  T1: 900MVA 20 kV-230 kV/RConn1 -- 25km Area 1/LConn1
  T1: 900MVA 20 kV-230 kV/RConn2 -- 25km Area 1/LConn2
  Snubber1/LConn1 -- Three-Phase V-I Measurement1/RConn1 -- T2: 900MVA 20 kV/230 kV/LConn1
  Snubber1/LConn2 -- T2: 900MVA 20 kV/230 kV/LConn2 -- Three-Phase V-I Measurement1/RConn2
  Snubber1/LConn3 -- T2: 900MVA 20 kV/230 kV/LConn3 -- Three-Phase V-I Measurement1/RConn3
  T1: 900MVA 20 kV-230 kV/RConn3 -- 25km Area 1/LConn3
  Snubber/LConn1 -- T1: 900MVA 20 kV-230 kV/LConn1 -- Three-Phase V-I Measurement/RConn1
  T1: 900MVA 20 kV-230 kV/LConn2 -- Three-Phase V-I Measurement/RConn2 -- Snubber/LConn2
  T1: 900MVA 20 kV-230 kV/LConn3 -- Three-Phase V-I Measurement/RConn3 -- Snubber/LConn3
  25km Area 1/RConn2 -- T2: 900MVA 20 kV/230 kV/RConn2 -- 10 km Area 1/LConn2
  25km Area 1/RConn1 -- T2: 900MVA 20 kV/230 kV/RConn1 -- 10 km Area 1/LConn1
  25km Area 1/RConn3 -- T2: 900MVA 20 kV/230 kV/RConn3 -- 10 km Area 1/LConn3
  10 km Area 1/RConn2 -- 2 MVA 420V / 230e3V/LConn2 -- " B"/RConn1 -- -200MVAR/LConn2 -- "800MW "/LConn2 -- "T1: 900MVA "/RConn2 -- 967MW 100MVAR -187MVAR/LConn2
  2 MVA 420V / 230e3V/RConn3 -- "BESS2 "/RConn3 -- BESS/RConn3
  2 MVA 420V / 230e3V/RConn2 -- "BESS2 "/RConn2 -- BESS/RConn2
  2 MVA 420V / 230e3V/RConn1 -- "BESS2 "/RConn1 -- BESS/RConn1
  Three-Phase V-I Measurement/LConn3 -- M1 900 MVA/RConn3
  Three-Phase V-I Measurement/LConn2 -- M1 900 MVA/RConn2
  Three-Phase V-I Measurement/LConn1 -- M1 900 MVA/RConn1
  Three-Phase V-I Measurement1/LConn1 -- M2 900 MVA/RConn1
  Three-Phase V-I Measurement1/LConn2 -- M2 900 MVA/RConn2
  Three-Phase V-I Measurement1/LConn3 -- M2 900 MVA/RConn3
  IEEE 13-node distribution feeder/LConn1 -- "T1: 900MVA "/LConn1
  IEEE 13-node distribution feeder/LConn2 -- "T1: 900MVA "/LConn2
  IEEE 13-node distribution feeder/LConn3 -- "T1: 900MVA "/LConn3
  10 km Area 1/RConn3 -- 2 MVA 420V / 230e3V/LConn3 -- " C"/RConn1 -- -200MVAR/LConn3 -- "800MW "/LConn3 -- "T1: 900MVA "/RConn3 -- 967MW 100MVAR -187MVAR/LConn3
  10 km Area 1/RConn1 -- 2 MVA 420V / 230e3V/LConn1 -- " A"/RConn1 -- -200MVAR/LConn1 -- "800MW "/LConn1 -- "T1: 900MVA "/RConn1 -- 967MW 100MVAR -187MVAR/LConn1
